simulink model "Lab_1_1_simulink_tutorial"  (R2019b)
settings: Solver=ode113  StartTime=0.0  StopTime=1000  MaxStep=0.01  RelTol=1e-13
settings Model: Creator=adity  LastModifiedBy=adity

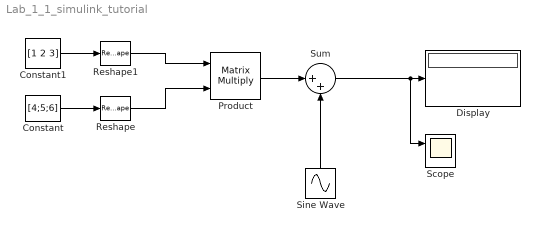
== system Lab_1_1_simulink_tutorial ==
  Constant : Constant  Value=[4;5;6]
  Constant1 : Constant  Value=[1 2 3]
  Display : Display
  Product : Product  Multiplication=Matrix(*)
  Reshape : Reshape  OutputDimensionality=Column vector (2-D)
  Reshape1 : Reshape  OutputDimensionality=Row vector (2-D)
  Scope : Scope  NumInputPorts=2
  Sine Wave : Sin  SampleTime=0
  Sum : Sum  Inputs=|++
  wires:
  Constant1/1 -> Reshape1/1
  Constant/1 -> Reshape/1
  Sum/1 -> Scope/1, Display/1
  Product/1 -> Sum/1
  Sine Wave/1 -> Sum/2
  Reshape/1 -> Product/2
  Reshape1/1 -> Product/1
